simulink model "sudoku"  (R2012b)
settings: Solver=ode45  StartTime=0.0  StopTime=10.0  RelTol=1e-3
libraries: sldvlib x83
(part 1 of 4)
settings Model: Creator=roberto  LastModifiedBy=roberto

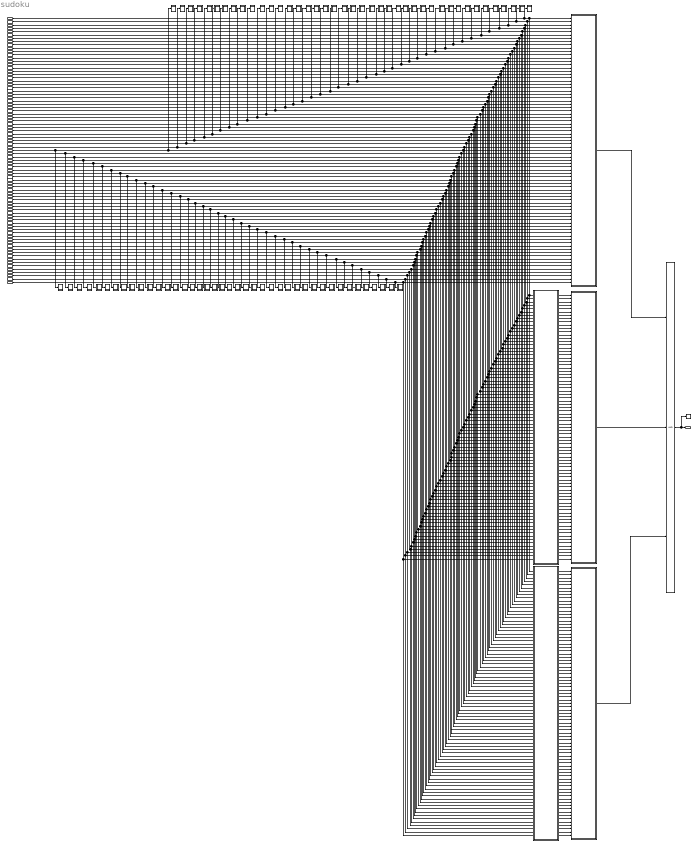
== system sudoku ==
  In1 : Inport  OutDataTypeStr=int8
  In2 : Inport  Port=2  OutDataTypeStr=int8
  In3 : Inport  Port=3  OutDataTypeStr=int8
  In4 : Inport  Port=4  OutDataTypeStr=int8
  In5 : Inport  Port=5  OutDataTypeStr=int8
  In6 : Inport  Port=6  OutDataTypeStr=int8
  In7 : Inport  Port=7  OutDataTypeStr=int8
  In8 : Inport  Port=8  OutDataTypeStr=int8
  In9 : Inport  Port=9  OutDataTypeStr=int8
  In10 : Inport  Port=10  OutDataTypeStr=int8
  In11 : Inport  Port=11  OutDataTypeStr=int8
  In12 : Inport  Port=12  OutDataTypeStr=int8
  In13 : Inport  Port=13  OutDataTypeStr=int8
  In14 : Inport  Port=14  OutDataTypeStr=int8
  In15 : Inport  Port=15  OutDataTypeStr=int8
  In16 : Inport  Port=16  OutDataTypeStr=int8
  In17 : Inport  Port=17  OutDataTypeStr=int8
  In18 : Inport  Port=18  OutDataTypeStr=int8
  In19 : Inport  Port=19  OutDataTypeStr=int8
  In20 : Inport  Port=20  OutDataTypeStr=int8
  In21 : Inport  Port=21  OutDataTypeStr=int8
  In22 : Inport  Port=22  OutDataTypeStr=int8
  In23 : Inport  Port=23  OutDataTypeStr=int8
  In24 : Inport  Port=24  OutDataTypeStr=int8
  In25 : Inport  Port=25  OutDataTypeStr=int8
  In26 : Inport  Port=26  OutDataTypeStr=int8
  In27 : Inport  Port=27  OutDataTypeStr=int8
  In28 : Inport  Port=28  OutDataTypeStr=int8
  In29 : Inport  Port=29  OutDataTypeStr=int8
  In30 : Inport  Port=30  OutDataTypeStr=int8
  In31 : Inport  Port=31  OutDataTypeStr=int8
  In32 : Inport  Port=32  OutDataTypeStr=int8
  In33 : Inport  Port=33  OutDataTypeStr=int8
  In34 : Inport  Port=34  OutDataTypeStr=int8
  In35 : Inport  Port=35  OutDataTypeStr=int8
  In36 : Inport  Port=36  OutDataTypeStr=int8
  In37 : Inport  Port=37  OutDataTypeStr=int8
  In38 : Inport  Port=38  OutDataTypeStr=int8
  In39 : Inport  Port=39  OutDataTypeStr=int8
  In40 : Inport  Port=40  OutDataTypeStr=int8
  In41 : Inport  Port=41  OutDataTypeStr=int8
  In42 : Inport  Port=42  OutDataTypeStr=int8
  In43 : Inport  Port=43  OutDataTypeStr=int8
  In44 : Inport  Port=44  OutDataTypeStr=int8
  In45 : Inport  Port=45  OutDataTypeStr=int8
  In46 : Inport  Port=46  OutDataTypeStr=int8
  In47 : Inport  Port=47  OutDataTypeStr=int8
  In48 : Inport  Port=48  OutDataTypeStr=int8
  In49 : Inport  Port=49  OutDataTypeStr=int8
  In50 : Inport  Port=50  OutDataTypeStr=int8
  In51 : Inport  Port=51  OutDataTypeStr=int8
  In52 : Inport  Port=52  OutDataTypeStr=int8
  In53 : Inport  Port=53  OutDataTypeStr=int8
  In54 : Inport  Port=54  OutDataTypeStr=int8
  In55 : Inport  Port=55  OutDataTypeStr=int8
  In56 : Inport  Port=56  OutDataTypeStr=int8
  In57 : Inport  Port=57  OutDataTypeStr=int8
  In58 : Inport  Port=58  OutDataTypeStr=int8
  In59 : Inport  Port=59  OutDataTypeStr=int8
  In60 : Inport  Port=60  OutDataTypeStr=int8
  In61 : Inport  Port=61  OutDataTypeStr=int8
  In62 : Inport  Port=62  OutDataTypeStr=int8
  In63 : Inport  Port=63  OutDataTypeStr=int8
  In64 : Inport  Port=64  OutDataTypeStr=int8
  In65 : Inport  Port=65  OutDataTypeStr=int8
  In66 : Inport  Port=66  OutDataTypeStr=int8
  In67 : Inport  Port=67  OutDataTypeStr=int8
  In68 : Inport  Port=68  OutDataTypeStr=int8
  In69 : Inport  Port=69  OutDataTypeStr=int8
  In70 : Inport  Port=70  OutDataTypeStr=int8
  In71 : Inport  Port=71  OutDataTypeStr=int8
  In72 : Inport  Port=72  OutDataTypeStr=int8
  In73 : Inport  Port=73  OutDataTypeStr=int8
  In74 : Inport  Port=74  OutDataTypeStr=int8
  In75 : Inport  Port=75  OutDataTypeStr=int8
  In76 : Inport  Port=76  OutDataTypeStr=int8
  In77 : Inport  Port=77  OutDataTypeStr=int8
  In78 : Inport  Port=78  OutDataTypeStr=int8
  In79 : Inport  Port=79  OutDataTypeStr=int8
  In80 : Inport  Port=80  OutDataTypeStr=int8
  In81 : Inport  Port=81  OutDataTypeStr=int8
  BlockRewire : Subsystem
  ColRewire : Subsystem
  Logical Operator : Logic  Inputs=3  AllPortsSameDT=off  OutDataTypeStr=boolean
  Proof Objective : sldvlib/Objectives and Constraints/Proof Objective  enabled=on  customAVTBlockType=Proof Objective  intervals=true  dispValues=on  outEnabled=on  enableStopSim=off
      settings: AttributesFormatString=%<intervals>
  Rows : Subsystem
  blocks : Subsystem
  bounds : Subsystem
  bounds1 : Subsystem
  bounds10 : Subsystem
  bounds11 : Subsystem
  bounds12 : Subsystem
  bounds13 : Subsystem
  bounds14 : Subsystem
  bounds15 : Subsystem
  bounds16 : Subsystem
  bounds17 : Subsystem
  bounds18 : Subsystem
  bounds19 : Subsystem
  bounds2 : Subsystem
  bounds20 : Subsystem
  bounds21 : Subsystem
  bounds22 : Subsystem
  bounds23 : Subsystem
  bounds24 : Subsystem
  bounds25 : Subsystem
  bounds26 : Subsystem
  bounds27 : Subsystem
  bounds28 : Subsystem
  bounds29 : Subsystem
  bounds3 : Subsystem
  bounds30 : Subsystem
  bounds31 : Subsystem
  bounds32 : Subsystem
  bounds33 : Subsystem
  bounds34 : Subsystem
  bounds35 : Subsystem
  bounds36 : Subsystem
  bounds37 : Subsystem
  bounds38 : Subsystem
  bounds39 : Subsystem
  bounds4 : Subsystem
  bounds40 : Subsystem
  bounds41 : Subsystem
  bounds42 : Subsystem
  bounds43 : Subsystem
  bounds44 : Subsystem
  bounds45 : Subsystem
  bounds46 : Subsystem
  bounds47 : Subsystem
  bounds48 : Subsystem
  bounds49 : Subsystem
  bounds5 : Subsystem
  bounds50 : Subsystem
  bounds51 : Subsystem
  bounds52 : Subsystem
  bounds53 : Subsystem
  bounds54 : Subsystem
  bounds55 : Subsystem
  bounds56 : Subsystem
  bounds57 : Subsystem
  bounds58 : Subsystem
  bounds59 : Subsystem
  bounds6 : Subsystem
  bounds60 : Subsystem
  bounds61 : Subsystem
  bounds62 : Subsystem
  bounds63 : Subsystem
  bounds64 : Subsystem
  bounds65 : Subsystem
  bounds66 : Subsystem
  bounds67 : Subsystem
  bounds68 : Subsystem
  bounds69 : Subsystem
  bounds7 : Subsystem
  bounds70 : Subsystem
  bounds71 : Subsystem
  bounds72 : Subsystem
  bounds73 : Subsystem
  bounds74 : Subsystem
  bounds75 : Subsystem
  bounds76 : Subsystem
  bounds77 : Subsystem
  bounds78 : Subsystem
  bounds79 : Subsystem
  bounds8 : Subsystem
  bounds80 : Subsystem
  bounds81 : Subsystem
  bounds9 : Subsystem
  columns : Subsystem
  Out1 : Outport
  wires:
  In2/1 -> bounds1/1(In1), BlockRewire/2(In2), ColRewire/2(In2), Rows/2(In2)
  In3/1 -> bounds2/1(In1), BlockRewire/3(In3), ColRewire/3(In3), Rows/3(In3)
  In4/1 -> bounds3/1(In1), BlockRewire/4(In4), ColRewire/4(In4), Rows/4(In4)
  In5/1 -> bounds4/1(In1), BlockRewire/5(In5), ColRewire/5(In5), Rows/5(In5)
  In6/1 -> bounds5/1(In1), BlockRewire/6(In6), ColRewire/6(In6), Rows/6(In6)
  In7/1 -> bounds6/1(In1), BlockRewire/7(In7), ColRewire/7(In7), Rows/7(In7)
  In8/1 -> bounds7/1(In1), BlockRewire/8(In8), ColRewire/8(In8), Rows/8(In8)
  In9/1 -> bounds8/1(In1), BlockRewire/9(In9), ColRewire/9(In9), Rows/9(In9)
  In10/1 -> bounds9/1(In1), BlockRewire/10(In10), ColRewire/10(In10), Rows/10(In10)
  In11/1 -> bounds10/1(In1), BlockRewire/11(In11), ColRewire/11(In11), Rows/11(In11)
  In12/1 -> bounds11/1(In1), BlockRewire/12(In12), ColRewire/12(In12), Rows/12(In12)
  In13/1 -> bounds12/1(In1), BlockRewire/13(In13), ColRewire/13(In13), Rows/13(In13)
  In14/1 -> bounds13/1(In1), BlockRewire/14(In14), ColRewire/14(In14), Rows/14(In14)
  In16/1 -> bounds15/1(In1), BlockRewire/16(In16), ColRewire/16(In16), Rows/16(In16)
  In17/1 -> bounds16/1(In1), BlockRewire/17(In17), ColRewire/17(In17), Rows/17(In17)
  In18/1 -> bounds17/1(In1), BlockRewire/18(In18), ColRewire/18(In18), Rows/18(In18)
  In19/1 -> bounds18/1(In1), BlockRewire/19(In19), ColRewire/19(In19), Rows/19(In19)
  In21/1 -> bounds20/1(In1), BlockRewire/21(In21), ColRewire/21(In21), Rows/21(In21)
  In22/1 -> bounds21/1(In1), BlockRewire/22(In22), ColRewire/22(In22), Rows/22(In22)
  In23/1 -> bounds22/1(In1), BlockRewire/23(In23), ColRewire/23(In23), Rows/23(In23)
  In24/1 -> bounds23/1(In1), BlockRewire/24(In24), ColRewire/24(In24), Rows/24(In24)
  In25/1 -> bounds24/1(In1), BlockRewire/25(In25), ColRewire/25(In25), Rows/25(In25)
  In26/1 -> bounds25/1(In1), BlockRewire/26(In26), ColRewire/26(In26), Rows/26(In26)
  In27/1 -> bounds26/1(In1), BlockRewire/27(In27), ColRewire/27(In27), Rows/27(In27)
  In28/1 -> bounds27/1(In1), BlockRewire/28(In28), ColRewire/28(In28), Rows/28(In28)
  In29/1 -> bounds28/1(In1), BlockRewire/29(In29), ColRewire/29(In29), Rows/29(In29)
  In30/1 -> bounds29/1(In1), BlockRewire/30(In30), ColRewire/30(In30), Rows/30(In30)
  In31/1 -> bounds30/1(In1), BlockRewire/31(In31), ColRewire/31(In31), Rows/31(In31)
  In33/1 -> bounds32/1(In1), BlockRewire/33(In33), ColRewire/33(In33), Rows/33(In33)
  In34/1 -> bounds33/1(In1), BlockRewire/34(In34), ColRewire/34(In34), Rows/34(In34)
  In35/1 -> bounds34/1(In1), BlockRewire/35(In35), ColRewire/35(In35), Rows/35(In35)
  In36/1 -> bounds35/1(In1), BlockRewire/36(In36), ColRewire/36(In36), Rows/36(In36)
  In38/1 -> bounds37/1(In1), BlockRewire/38(In38), ColRewire/38(In38), Rows/38(In38)
  In39/1 -> bounds38/1(In1), BlockRewire/39(In39), ColRewire/39(In39), Rows/39(In39)
  In40/1 -> bounds39/1(In1), BlockRewire/40(In40), ColRewire/40(In40), Rows/40(In40)
  In42/1 -> bounds43/1(In1), BlockRewire/42(In42), ColRewire/42(In42), Rows/42(In42)
  In43/1 -> bounds44/1(In1), BlockRewire/43(In43), ColRewire/43(In43), Rows/43(In43)
  In44/1 -> bounds45/1(In1), BlockRewire/44(In44), ColRewire/44(In44), Rows/44(In44)
  In45/1 -> bounds46/1(In1), BlockRewire/45(In45), ColRewire/45(In45), Rows/45(In45)
  In46/1 -> bounds47/1(In1), BlockRewire/46(In46), ColRewire/46(In46), Rows/46(In46)
  In47/1 -> bounds48/1(In1), BlockRewire/47(In47), ColRewire/47(In47), Rows/47(In47)
  In48/1 -> bounds49/1(In1), BlockRewire/48(In48), ColRewire/48(In48), Rows/48(In48)
  In49/1 -> bounds50/1(In1), BlockRewire/49(In49), ColRewire/49(In49), Rows/49(In49)
  In50/1 -> bounds51/1(In1), BlockRewire/50(In50), ColRewire/50(In50), Rows/50(In50)
  In51/1 -> bounds52/1(In1), BlockRewire/51(In51), ColRewire/51(In51), Rows/51(In51)
  In52/1 -> bounds53/1(In1), BlockRewire/52(In52), ColRewire/52(In52), Rows/52(In52)
  In53/1 -> bounds54/1(In1), BlockRewire/53(In53), ColRewire/53(In53), Rows/53(In53)
  In54/1 -> bounds55/1(In1), BlockRewire/54(In54), ColRewire/54(In54), Rows/54(In54)
  In55/1 -> bounds56/1(In1), BlockRewire/55(In55), ColRewire/55(In55), Rows/55(In55)
  In56/1 -> bounds57/1(In1), BlockRewire/56(In56), ColRewire/56(In56), Rows/56(In56)
  In57/1 -> bounds58/1(In1), BlockRewire/57(In57), ColRewire/57(In57), Rows/57(In57)
  In58/1 -> bounds59/1(In1), BlockRewire/58(In58), ColRewire/58(In58), Rows/58(In58)
  In59/1 -> bounds60/1(In1), BlockRewire/59(In59), ColRewire/59(In59), Rows/59(In59)
  In60/1 -> bounds61/1(In1), BlockRewire/60(In60), ColRewire/60(In60), Rows/60(In60)
  In61/1 -> bounds62/1(In1), BlockRewire/61(In61), ColRewire/61(In61), Rows/61(In61)
  In62/1 -> bounds63/1(In1), BlockRewire/62(In62), ColRewire/62(In62), Rows/62(In62)
  In63/1 -> bounds64/1(In1), ColRewire/63(In63), BlockRewire/63(In63), Rows/63(In63)
  In64/1 -> bounds65/1(In1), BlockRewire/64(In64), ColRewire/64(In64), Rows/64(In64)
  In66/1 -> bounds67/1(In1), BlockRewire/66(In66), ColRewire/66(In66), Rows/66(In66)
  In68/1 -> bounds69/1(In1), BlockRewire/68(In68), ColRewire/68(In68), Rows/68(In68)
  In70/1 -> bounds71/1(In1), BlockRewire/70(In70), ColRewire/70(In70), Rows/70(In70)
  In71/1 -> bounds72/1(In1), BlockRewire/71(In71), ColRewire/71(In71), Rows/71(In71)
  In72/1 -> bounds73/1(In1), BlockRewire/72(In72), ColRewire/72(In72), Rows/72(In72)
  In74/1 -> bounds75/1(In1), BlockRewire/74(In74), ColRewire/74(In74), Rows/74(In74)
  In75/1 -> bounds76/1(In1), BlockRewire/75(In75), ColRewire/75(In75), Rows/75(In75)
  In76/1 -> bounds77/1(In1), BlockRewire/76(In76), ColRewire/76(In76), Rows/76(In76)
  In77/1 -> bounds78/1(In1), BlockRewire/77(In77), ColRewire/77(In77), Rows/77(In77)
  In78/1 -> bounds79/1(In1), BlockRewire/78(In78), ColRewire/78(In78), Rows/78(In78)
  In79/1 -> bounds80/1(In1), BlockRewire/79(In79), ColRewire/79(In79), Rows/79(In79)
  In80/1 -> bounds81/1(In1), BlockRewire/80(In80), ColRewire/80(In80), Rows/80(In80)
  In81/1 -> bounds41/1(In1), BlockRewire/81(In81), ColRewire/81(In81), Rows/81(In81)
  In69/1 -> bounds70/1(In1), BlockRewire/69(In69), ColRewire/69(In69), Rows/69(In69)
  In73/1 -> bounds74/1(In1), BlockRewire/73(In73), ColRewire/73(In73), Rows/73(In73)
  ColRewire/1(Out1) -> columns/1(In1)
  ColRewire/2(Out2) -> columns/2(In2)
  ColRewire/3(Out3) -> columns/3(In3)
  ColRewire/4(Out4) -> columns/4(In4)
  ColRewire/5(Out5) -> columns/5(In5)
  ColRewire/6(Out6) -> columns/6(In6)
  ColRewire/7(Out7) -> columns/7(In7)
  ColRewire/8(Out8) -> columns/8(In8)
  ColRewire/9(Out9) -> columns/9(In9)
  ColRewire/10(Out10) -> columns/10(In10)
  ColRewire/11(Out11) -> columns/11(In11)
  ColRewire/12(Out12) -> columns/12(In12)
  ColRewire/13(Out13) -> columns/13(In13)
  ColRewire/14(Out14) -> columns/14(In14)
  ColRewire/15(Out15) -> columns/15(In15)
  ColRewire/16(Out16) -> columns/16(In16)
  ColRewire/17(Out17) -> columns/17(In17)
  ColRewire/18(Out18) -> columns/18(In18)
  ColRewire/19(Out19) -> columns/19(In19)
  ColRewire/20(Out20) -> columns/20(In20)
  ColRewire/21(Out21) -> columns/21(In21)
  ColRewire/22(Out22) -> columns/22(In22)
  ColRewire/23(Out23) -> columns/23(In23)
  ColRewire/24(Out24) -> columns/24(In24)
  ColRewire/25(Out25) -> columns/25(In25)
  ColRewire/26(Out26) -> columns/26(In26)
  ColRewire/27(Out27) -> columns/27(In27)
  ColRewire/28(Out28) -> columns/28(In28)
  ColRewire/29(Out29) -> columns/29(In29)
  ColRewire/30(Out30) -> columns/30(In30)
  ColRewire/31(Out31) -> columns/31(In31)
  ColRewire/32(Out32) -> columns/32(In32)
  ColRewire/33(Out33) -> columns/33(In33)
  ColRewire/34(Out34) -> columns/34(In34)
  ColRewire/35(Out35) -> columns/35(In35)
  ColRewire/36(Out36) -> columns/36(In36)
  ColRewire/37(Out37) -> columns/37(In37)
  ColRewire/38(Out38) -> columns/38(In38)
  ColRewire/39(Out39) -> columns/39(In39)
  ColRewire/40(Out40) -> columns/40(In40)
  ColRewire/41(Out41) -> columns/41(In41)
  ColRewire/42(Out42) -> columns/42(In42)
  ColRewire/43(Out43) -> columns/43(In43)
  ColRewire/44(Out44) -> columns/44(In44)
  ColRewire/45(Out45) -> columns/45(In45)
  ColRewire/46(Out46) -> columns/46(In46)
  ColRewire/47(Out47) -> columns/47(In47)
  ColRewire/48(Out48) -> columns/48(In48)
  ColRewire/49(Out49) -> columns/49(In49)
  ColRewire/50(Out50) -> columns/50(In50)
  ColRewire/51(Out51) -> columns/51(In51)
  ColRewire/52(Out52) -> columns/52(In52)
  ColRewire/53(Out53) -> columns/53(In53)
  ColRewire/54(Out54) -> columns/54(In54)
  ColRewire/55(Out55) -> columns/55(In55)
  ColRewire/56(Out56) -> columns/56(In56)
  ColRewire/57(Out57) -> columns/57(In57)
  ColRewire/58(Out58) -> columns/58(In58)
  ColRewire/59(Out59) -> columns/59(In59)
  ColRewire/60(Out60) -> columns/60(In60)
  ColRewire/61(Out61) -> columns/61(In61)
  ColRewire/62(Out62) -> columns/62(In62)
  ColRewire/63(Out63) -> columns/63(In63)
  ColRewire/64(Out64) -> columns/64(In64)
  ColRewire/65(Out65) -> columns/65(In65)
  ColRewire/66(Out66) -> columns/66(In66)
  ColRewire/67(Out67) -> columns/67(In67)
  ColRewire/68(Out68) -> columns/68(In68)
  ColRewire/70(Out70) -> columns/70(In70)
  ColRewire/71(Out71) -> columns/71(In71)
  ColRewire/72(Out72) -> columns/72(In72)
  ColRewire/74(Out74) -> columns/74(In74)
  ColRewire/75(Out75) -> columns/75(In75)
  ColRewire/76(Out76) -> columns/76(In76)
  ColRewire/77(Out77) -> columns/77(In77)
  ColRewire/78(Out78) -> columns/78(In78)
  ColRewire/79(Out79) -> columns/79(In79)
  ColRewire/80(Out80) -> columns/80(In80)
  ColRewire/81(Out81) -> columns/81(In81)
  ColRewire/69(Out69) -> columns/69(In69)
  ColRewire/73(Out73) -> columns/73(In73)
  BlockRewire/1(Out1) -> blocks/1(In1)
  BlockRewire/2(Out10) -> blocks/2(In2)
  BlockRewire/3(Out19) -> blocks/3(In3)
  BlockRewire/4(Out2) -> blocks/4(In4)
  BlockRewire/5(Out11) -> blocks/5(In5)
  BlockRewire/6(Out20) -> blocks/6(In6)
  BlockRewire/7(Out3) -> blocks/7(In7)
  BlockRewire/8(Out12) -> blocks/8(In8)
  BlockRewire/9(Out21) -> blocks/9(In9)
  BlockRewire/10(Out28) -> blocks/10(In10)
  BlockRewire/11(Out37) -> blocks/11(In11)
  BlockRewire/12(Out46) -> blocks/12(In12)
  BlockRewire/13(Out29) -> blocks/13(In13)
  BlockRewire/15(Out47) -> blocks/15(In15)
  BlockRewire/16(Out30) -> blocks/16(In16)
  BlockRewire/17(Out39) -> blocks/17(In17)
  BlockRewire/18(Out48) -> blocks/18(In18)
  BlockRewire/19(Out55) -> blocks/19(In19)
  BlockRewire/20(Out64) -> blocks/20(In20)
  BlockRewire/21(Out73) -> blocks/21(In21)
  BlockRewire/22(Out56) -> blocks/22(In22)
  BlockRewire/23(Out65) -> blocks/23(In23)
  BlockRewire/24(Out74) -> blocks/24(In24)
  BlockRewire/25(Out57) -> blocks/25(In25)
  BlockRewire/26(Out66) -> blocks/26(In26)
  BlockRewire/27(Out75) -> blocks/27(In27)
  BlockRewire/28(Out4) -> blocks/28(In28)
  BlockRewire/29(Out13) -> blocks/29(In29)
  BlockRewire/30(Out22) -> blocks/30(In30)
  BlockRewire/31(Out5) -> blocks/31(In31)
  BlockRewire/32(Out14) -> blocks/32(In32)
  BlockRewire/33(Out23) -> blocks/33(In33)
  BlockRewire/34(Out6) -> blocks/34(In34)
  BlockRewire/35(Out15) -> blocks/35(In35)
  BlockRewire/36(Out24) -> blocks/36(In36)
  BlockRewire/37(Out31) -> blocks/37(In37)
  BlockRewire/38(Out40) -> blocks/38(In38)
  BlockRewire/39(Out49) -> blocks/39(In39)
  BlockRewire/40(Out32) -> blocks/40(In40)
  BlockRewire/41(Out41) -> blocks/41(In41)
  BlockRewire/42(Out50) -> blocks/42(In42)
  BlockRewire/43(Out33) -> blocks/43(In43)
  BlockRewire/44(Out42) -> blocks/44(In44)
  BlockRewire/45(Out51) -> blocks/45(In45)
  BlockRewire/46(Out58) -> blocks/46(In46)
  BlockRewire/47(Out67) -> blocks/47(In47)
  BlockRewire/48(Out76) -> blocks/48(In48)
  BlockRewire/49(Out59) -> blocks/49(In49)
  BlockRewire/50(Out68) -> blocks/50(In50)
  BlockRewire/51(Out77) -> blocks/51(In51)
  BlockRewire/52(Out60) -> blocks/52(In52)
  BlockRewire/53(Out69) -> blocks/53(In53)
  BlockRewire/54(Out78) -> blocks/54(In54)
  BlockRewire/55(Out7) -> blocks/55(In55)
  BlockRewire/56(Out16) -> blocks/56(In56)
  BlockRewire/57(Out25) -> blocks/57(In57)
  BlockRewire/58(Out8) -> blocks/58(In58)
  BlockRewire/59(Out17) -> blocks/59(In59)
  BlockRewire/60(Out26) -> blocks/60(In60)
  BlockRewire/61(Out9) -> blocks/61(In61)
  BlockRewire/62(Out18) -> blocks/62(In62)
  BlockRewire/63(Out27) -> blocks/63(In63)
  BlockRewire/64(Out34) -> blocks/64(In64)
  BlockRewire/65(Out43) -> blocks/65(In65)
  BlockRewire/66(Out52) -> blocks/66(In66)
  BlockRewire/67(Out35) -> blocks/67(In67)
  BlockRewire/68(Out44) -> blocks/68(In68)
  BlockRewire/69(Out53) -> blocks/69(In69)
  BlockRewire/70(Out36) -> blocks/70(In70)
  BlockRewire/71(Out45) -> blocks/71(In71)
  BlockRewire/72(Out54) -> blocks/72(In72)
  BlockRewire/73(Out61) -> blocks/73(In73)
  BlockRewire/74(Out70) -> blocks/74(In74)
  BlockRewire/75(Out79) -> blocks/75(In75)
  BlockRewire/76(Out62) -> blocks/76(In76)
  BlockRewire/77(Out71) -> blocks/77(In77)
  BlockRewire/78(Out80) -> blocks/78(In78)
  BlockRewire/79(Out63) -> blocks/79(In79)
  BlockRewire/80(Out72) -> blocks/80(In80)
  BlockRewire/81(Out81) -> blocks/81(In81)
  In15/1 -> bounds14/1(In1), BlockRewire/15(In15), ColRewire/15(In15), Rows/15(In15)
  In32/1 -> bounds31/1(In1), BlockRewire/32(In32), ColRewire/32(In32), Rows/32(In32)
  In37/1 -> bounds36/1(In1), BlockRewire/37(In37), ColRewire/37(In37), Rows/37(In37)
  In41/1 -> bounds42/1(In1), bounds40/1(In1), BlockRewire/41(In41), ColRewire/41(In41), Rows/41(In41)
  In65/1 -> bounds66/1(In1), ColRewire/65(In65), BlockRewire/65(In65), Rows/65(In65)
  BlockRewire/14(Out38) -> blocks/14(In14)
  In1/1 -> bounds/1(In1), BlockRewire/1(In1), ColRewire/1(In1), Rows/1(In1)
  In20/1 -> bounds19/1(In1), BlockRewire/20(In20), ColRewire/20(In20), Rows/20(In20)
  In67/1 -> bounds68/1(In1), BlockRewire/67(In67), ColRewire/67(In67), Rows/67(In67)
  Rows/1(Out1) -> Logical Operator/1
  columns/1(Out1) -> Logical Operator/2
  blocks/1(Out1) -> Logical Operator/3
  Logical Operator/1 -> Proof Objective/1, Out1/1

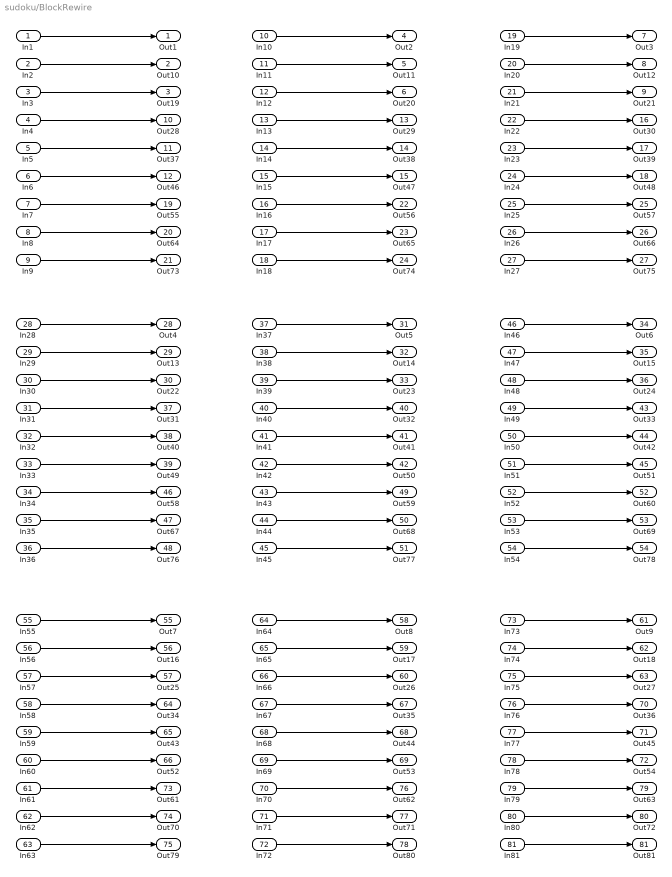
== system sudoku/BlockRewire ==
  In1 : Inport
  In2 : Inport  Port=2
  In3 : Inport  Port=3
  In4 : Inport  Port=4
  In5 : Inport  Port=5
  In6 : Inport  Port=6
  In7 : Inport  Port=7
  In8 : Inport  Port=8
  In9 : Inport  Port=9
  In10 : Inport  Port=10
  In11 : Inport  Port=11
  In12 : Inport  Port=12
  In13 : Inport  Port=13
  In14 : Inport  Port=14
  In15 : Inport  Port=15
  In16 : Inport  Port=16
  In17 : Inport  Port=17
  In18 : Inport  Port=18
  In19 : Inport  Port=19
  In20 : Inport  Port=20
  In21 : Inport  Port=21
  In22 : Inport  Port=22
  In23 : Inport  Port=23
  In24 : Inport  Port=24
  In25 : Inport  Port=25
  In26 : Inport  Port=26
  In27 : Inport  Port=27
  In28 : Inport  Port=28
  In29 : Inport  Port=29
  In30 : Inport  Port=30
  In31 : Inport  Port=31
  In32 : Inport  Port=32
  In33 : Inport  Port=33
  In34 : Inport  Port=34
  In35 : Inport  Port=35
  In36 : Inport  Port=36
  In37 : Inport  Port=37
  In38 : Inport  Port=38
  In39 : Inport  Port=39
  In40 : Inport  Port=40
  In41 : Inport  Port=41
  In42 : Inport  Port=42
  In43 : Inport  Port=43
  In44 : Inport  Port=44
  In45 : Inport  Port=45
  In46 : Inport  Port=46
  In47 : Inport  Port=47
  In48 : Inport  Port=48
  In49 : Inport  Port=49
  In50 : Inport  Port=50
  In51 : Inport  Port=51
  In52 : Inport  Port=52
  In53 : Inport  Port=53
  In54 : Inport  Port=54
  In55 : Inport  Port=55
  In56 : Inport  Port=56
  In57 : Inport  Port=57
  In58 : Inport  Port=58
  In59 : Inport  Port=59
  In60 : Inport  Port=60
  In61 : Inport  Port=61
  In62 : Inport  Port=62
  In63 : Inport  Port=63
  In64 : Inport  Port=64
  In65 : Inport  Port=65
  In66 : Inport  Port=66
  In67 : Inport  Port=67
  In68 : Inport  Port=68
  In69 : Inport  Port=69
  In70 : Inport  Port=70
  In71 : Inport  Port=71
  In72 : Inport  Port=72
  In73 : Inport  Port=73
  In74 : Inport  Port=74
  In75 : Inport  Port=75
  In76 : Inport  Port=76
  In77 : Inport  Port=77
  In78 : Inport  Port=78
  In79 : Inport  Port=79
  In80 : Inport  Port=80
  In81 : Inport  Port=81
  Out1 : Outport
  Out10 : Outport  Port=2
  Out19 : Outport  Port=3
  Out2 : Outport  Port=4
  Out11 : Outport  Port=5
  Out20 : Outport  Port=6
  Out3 : Outport  Port=7
  Out12 : Outport  Port=8
  Out21 : Outport  Port=9
  Out28 : Outport  Port=10
  Out37 : Outport  Port=11
  Out46 : Outport  Port=12
  Out29 : Outport  Port=13
  Out38 : Outport  Port=14
  Out47 : Outport  Port=15
  Out30 : Outport  Port=16
  Out39 : Outport  Port=17
  Out48 : Outport  Port=18
  Out55 : Outport  Port=19
  Out64 : Outport  Port=20
  Out73 : Outport  Port=21
  Out56 : Outport  Port=22
  Out65 : Outport  Port=23
  Out74 : Outport  Port=24
  Out57 : Outport  Port=25
  Out66 : Outport  Port=26
  Out75 : Outport  Port=27
  Out4 : Outport  Port=28
  Out13 : Outport  Port=29
  Out22 : Outport  Port=30
  Out5 : Outport  Port=31
  Out14 : Outport  Port=32
  Out23 : Outport  Port=33
  Out6 : Outport  Port=34
  Out15 : Outport  Port=35
  Out24 : Outport  Port=36
  Out31 : Outport  Port=37
  Out40 : Outport  Port=38
  Out49 : Outport  Port=39
  Out32 : Outport  Port=40
  Out41 : Outport  Port=41
  Out50 : Outport  Port=42
  Out33 : Outport  Port=43
  Out42 : Outport  Port=44
  Out51 : Outport  Port=45
  Out58 : Outport  Port=46
  Out67 : Outport  Port=47
  Out76 : Outport  Port=48
  Out59 : Outport  Port=49
  Out68 : Outport  Port=50
  Out77 : Outport  Port=51
  Out60 : Outport  Port=52
  Out69 : Outport  Port=53
  Out78 : Outport  Port=54
  Out7 : Outport  Port=55
  Out16 : Outport  Port=56
  Out25 : Outport  Port=57
  Out8 : Outport  Port=58
  Out17 : Outport  Port=59
  Out26 : Outport  Port=60
  Out9 : Outport  Port=61
  Out18 : Outport  Port=62
  Out27 : Outport  Port=63
  Out34 : Outport  Port=64
  Out43 : Outport  Port=65
  Out52 : Outport  Port=66
  Out35 : Outport  Port=67
  Out44 : Outport  Port=68
  Out53 : Outport  Port=69
  Out36 : Outport  Port=70
  Out45 : Outport  Port=71
  Out54 : Outport  Port=72
  Out61 : Outport  Port=73
  Out70 : Outport  Port=74
  Out79 : Outport  Port=75
  Out62 : Outport  Port=76
  Out71 : Outport  Port=77
  Out80 : Outport  Port=78
  Out63 : Outport  Port=79
  Out72 : Outport  Port=80
  Out81 : Outport  Port=81
  wires:
  In1/1 -> Out1/1
  In10/1 -> Out2/1
  In19/1 -> Out3/1
  In2/1 -> Out10/1
  In3/1 -> Out19/1
  In4/1 -> Out28/1
  In5/1 -> Out37/1
  In6/1 -> Out46/1
  In7/1 -> Out55/1
  In8/1 -> Out64/1
  In9/1 -> Out73/1
  In11/1 -> Out11/1
  In12/1 -> Out20/1
  In13/1 -> Out29/1
  In14/1 -> Out38/1
  In15/1 -> Out47/1
  In16/1 -> Out56/1
  In17/1 -> Out65/1
  In18/1 -> Out74/1
  In20/1 -> Out12/1
  In21/1 -> Out21/1
  In22/1 -> Out30/1
  In23/1 -> Out39/1
  In24/1 -> Out48/1
  In25/1 -> Out57/1
  In26/1 -> Out66/1
  In27/1 -> Out75/1
  In28/1 -> Out4/1
  In29/1 -> Out13/1
  In37/1 -> Out5/1
  In38/1 -> Out14/1
  In46/1 -> Out6/1
  In47/1 -> Out15/1
  In55/1 -> Out7/1
  In56/1 -> Out16/1
  In64/1 -> Out8/1
  In65/1 -> Out17/1
  In73/1 -> Out9/1
  In74/1 -> Out18/1
  In30/1 -> Out22/1
  In31/1 -> Out31/1
  In32/1 -> Out40/1
  In39/1 -> Out23/1
  In40/1 -> Out32/1
  In41/1 -> Out41/1
  In48/1 -> Out24/1
  In49/1 -> Out33/1
  In57/1 -> Out25/1
  In58/1 -> Out34/1
  In66/1 -> Out26/1
  In67/1 -> Out35/1
  In75/1 -> Out27/1
  In76/1 -> Out36/1
  In33/1 -> Out49/1
  In34/1 -> Out58/1
  In35/1 -> Out67/1
  In36/1 -> Out76/1
  In42/1 -> Out50/1
  In43/1 -> Out59/1
  In44/1 -> Out68/1
  In45/1 -> Out77/1
  In50/1 -> Out42/1
  In51/1 -> Out51/1
  In52/1 -> Out60/1
  In53/1 -> Out69/1
  In54/1 -> Out78/1
  In59/1 -> Out43/1
  In60/1 -> Out52/1
  In61/1 -> Out61/1
  In62/1 -> Out70/1
  In63/1 -> Out79/1
  In68/1 -> Out44/1
  In69/1 -> Out53/1
  In70/1 -> Out62/1
  In71/1 -> Out71/1
  In72/1 -> Out80/1
  In77/1 -> Out45/1
  In78/1 -> Out54/1
  In79/1 -> Out63/1
  In80/1 -> Out72/1
  In81/1 -> Out81/1

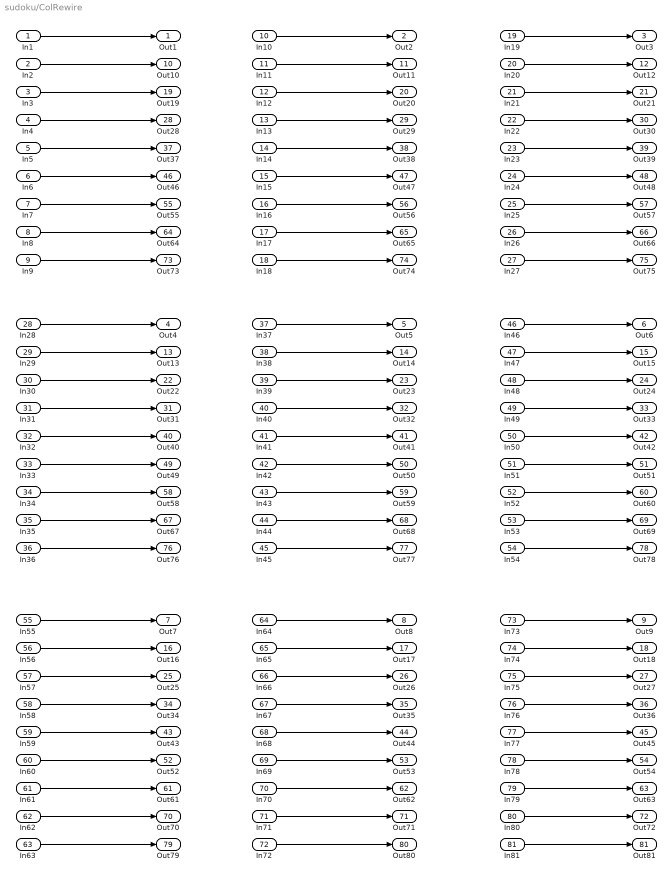
== system sudoku/ColRewire ==
  In1 : Inport
  In2 : Inport  Port=2
  In3 : Inport  Port=3
  In4 : Inport  Port=4
  In5 : Inport  Port=5
  In6 : Inport  Port=6
  In7 : Inport  Port=7
  In8 : Inport  Port=8
  In9 : Inport  Port=9
  In10 : Inport  Port=10
  In11 : Inport  Port=11
  In12 : Inport  Port=12
  In13 : Inport  Port=13
  In14 : Inport  Port=14
  In15 : Inport  Port=15
  In16 : Inport  Port=16
  In17 : Inport  Port=17
  In18 : Inport  Port=18
  In19 : Inport  Port=19
  In20 : Inport  Port=20
  In21 : Inport  Port=21
  In22 : Inport  Port=22
  In23 : Inport  Port=23
  In24 : Inport  Port=24
  In25 : Inport  Port=25
  In26 : Inport  Port=26
  In27 : Inport  Port=27
  In28 : Inport  Port=28
  In29 : Inport  Port=29
  In30 : Inport  Port=30
  In31 : Inport  Port=31
  In32 : Inport  Port=32
  In33 : Inport  Port=33
  In34 : Inport  Port=34
  In35 : Inport  Port=35
  In36 : Inport  Port=36
  In37 : Inport  Port=37
  In38 : Inport  Port=38
  In39 : Inport  Port=39
  In40 : Inport  Port=40
  In41 : Inport  Port=41
  In42 : Inport  Port=42
  In43 : Inport  Port=43
  In44 : Inport  Port=44
  In45 : Inport  Port=45
  In46 : Inport  Port=46
  In47 : Inport  Port=47
  In48 : Inport  Port=48
  In49 : Inport  Port=49
  In50 : Inport  Port=50
  In51 : Inport  Port=51
  In52 : Inport  Port=52
  In53 : Inport  Port=53
  In54 : Inport  Port=54
  In55 : Inport  Port=55
  In56 : Inport  Port=56
  In57 : Inport  Port=57
  In58 : Inport  Port=58
  In59 : Inport  Port=59
  In60 : Inport  Port=60
  In61 : Inport  Port=61
  In62 : Inport  Port=62
  In63 : Inport  Port=63
  In64 : Inport  Port=64
  In65 : Inport  Port=65
  In66 : Inport  Port=66
  In67 : Inport  Port=67
  In68 : Inport  Port=68
  In69 : Inport  Port=69
  In70 : Inport  Port=70
  In71 : Inport  Port=71
  In72 : Inport  Port=72
  In73 : Inport  Port=73
  In74 : Inport  Port=74
  In75 : Inport  Port=75
  In76 : Inport  Port=76
  In77 : Inport  Port=77
  In78 : Inport  Port=78
  In79 : Inport  Port=79
  In80 : Inport  Port=80
  In81 : Inport  Port=81
  Out1 : Outport
  Out2 : Outport  Port=2
  Out3 : Outport  Port=3
  Out4 : Outport  Port=4
  Out5 : Outport  Port=5
  Out6 : Outport  Port=6
  Out7 : Outport  Port=7
  Out8 : Outport  Port=8
  Out9 : Outport  Port=9
  Out10 : Outport  Port=10
  Out11 : Outport  Port=11
  Out12 : Outport  Port=12
  Out13 : Outport  Port=13
  Out14 : Outport  Port=14
  Out15 : Outport  Port=15
  Out16 : Outport  Port=16
  Out17 : Outport  Port=17
  Out18 : Outport  Port=18
  Out19 : Outport  Port=19
  Out20 : Outport  Port=20
  Out21 : Outport  Port=21
  Out22 : Outport  Port=22
  Out23 : Outport  Port=23
  Out24 : Outport  Port=24
  Out25 : Outport  Port=25
  Out26 : Outport  Port=26
  Out27 : Outport  Port=27
  Out28 : Outport  Port=28
  Out29 : Outport  Port=29
  Out30 : Outport  Port=30
  Out31 : Outport  Port=31
  Out32 : Outport  Port=32
  Out33 : Outport  Port=33
  Out34 : Outport  Port=34
  Out35 : Outport  Port=35
  Out36 : Outport  Port=36
  Out37 : Outport  Port=37
  Out38 : Outport  Port=38
  Out39 : Outport  Port=39
  Out40 : Outport  Port=40
  Out41 : Outport  Port=41
  Out42 : Outport  Port=42
  Out43 : Outport  Port=43
  Out44 : Outport  Port=44
  Out45 : Outport  Port=45
  Out46 : Outport  Port=46
  Out47 : Outport  Port=47
  Out48 : Outport  Port=48
  Out49 : Outport  Port=49
  Out50 : Outport  Port=50
  Out51 : Outport  Port=51
  Out52 : Outport  Port=52
  Out53 : Outport  Port=53
  Out54 : Outport  Port=54
  Out55 : Outport  Port=55
  Out56 : Outport  Port=56
  Out57 : Outport  Port=57
  Out58 : Outport  Port=58
  Out59 : Outport  Port=59
  Out60 : Outport  Port=60
  Out61 : Outport  Port=61
  Out62 : Outport  Port=62
  Out63 : Outport  Port=63
  Out64 : Outport  Port=64
  Out65 : Outport  Port=65
  Out66 : Outport  Port=66
  Out67 : Outport  Port=67
  Out68 : Outport  Port=68
  Out69 : Outport  Port=69
  Out70 : Outport  Port=70
  Out71 : Outport  Port=71
  Out72 : Outport  Port=72
  Out73 : Outport  Port=73
  Out74 : Outport  Port=74
  Out75 : Outport  Port=75
  Out76 : Outport  Port=76
  Out77 : Outport  Port=77
  Out78 : Outport  Port=78
  Out79 : Outport  Port=79
  Out80 : Outport  Port=80
  Out81 : Outport  Port=81
  wires:
  In1/1 -> Out1/1
  In10/1 -> Out2/1
  In19/1 -> Out3/1
  In2/1 -> Out10/1
  In3/1 -> Out19/1
  In4/1 -> Out28/1
  In5/1 -> Out37/1
  In6/1 -> Out46/1
  In7/1 -> Out55/1
  In8/1 -> Out64/1
  In9/1 -> Out73/1
  In11/1 -> Out11/1
  In12/1 -> Out20/1
  In13/1 -> Out29/1
  In14/1 -> Out38/1
  In15/1 -> Out47/1
  In16/1 -> Out56/1
  In17/1 -> Out65/1
  In18/1 -> Out74/1
  In20/1 -> Out12/1
  In21/1 -> Out21/1
  In22/1 -> Out30/1
  In23/1 -> Out39/1
  In24/1 -> Out48/1
  In25/1 -> Out57/1
  In26/1 -> Out66/1
  In27/1 -> Out75/1
  In28/1 -> Out4/1
  In29/1 -> Out13/1
  In37/1 -> Out5/1
  In38/1 -> Out14/1
  In46/1 -> Out6/1
  In47/1 -> Out15/1
  In55/1 -> Out7/1
  In56/1 -> Out16/1
  In64/1 -> Out8/1
  In65/1 -> Out17/1
  In73/1 -> Out9/1
  In74/1 -> Out18/1
  In30/1 -> Out22/1
  In31/1 -> Out31/1
  In32/1 -> Out40/1
  In39/1 -> Out23/1
  In40/1 -> Out32/1
  In41/1 -> Out41/1
  In48/1 -> Out24/1
  In49/1 -> Out33/1
  In57/1 -> Out25/1
  In58/1 -> Out34/1
  In66/1 -> Out26/1
  In67/1 -> Out35/1
  In75/1 -> Out27/1
  In76/1 -> Out36/1
  In33/1 -> Out49/1
  In34/1 -> Out58/1
  In35/1 -> Out67/1
  In36/1 -> Out76/1
  In42/1 -> Out50/1
  In43/1 -> Out59/1
  In44/1 -> Out68/1
  In45/1 -> Out77/1
  In50/1 -> Out42/1
  In51/1 -> Out51/1
  In52/1 -> Out60/1
  In53/1 -> Out69/1
  In54/1 -> Out78/1
  In59/1 -> Out43/1
  In60/1 -> Out52/1
  In61/1 -> Out61/1
  In62/1 -> Out70/1
  In63/1 -> Out79/1
  In68/1 -> Out44/1
  In69/1 -> Out53/1
  In70/1 -> Out62/1
  In71/1 -> Out71/1
  In72/1 -> Out80/1
  In77/1 -> Out45/1
  In78/1 -> Out54/1
  In79/1 -> Out63/1
  In80/1 -> Out72/1
  In81/1 -> Out81/1

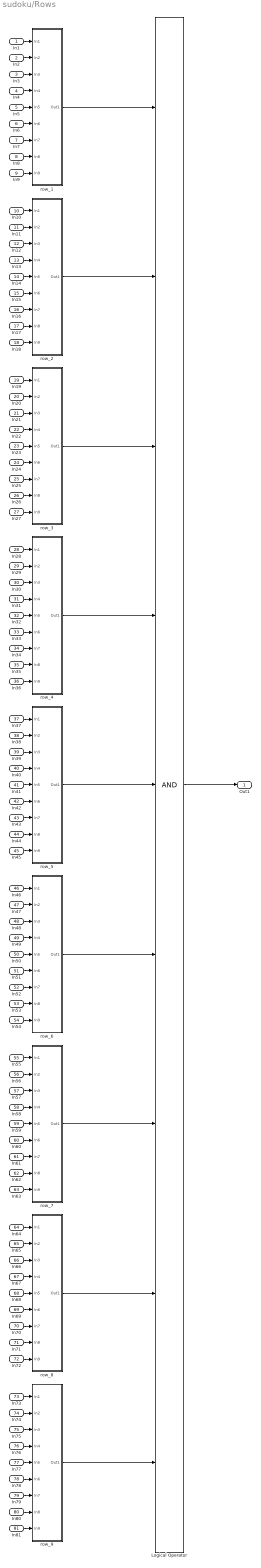
== system sudoku/Rows ==
  In1 : Inport
  In2 : Inport  Port=2
  In3 : Inport  Port=3
  In4 : Inport  Port=4
  In5 : Inport  Port=5
  In6 : Inport  Port=6
  In7 : Inport  Port=7
  In8 : Inport  Port=8
  In9 : Inport  Port=9
  In10 : Inport  Port=10
  In11 : Inport  Port=11
  In12 : Inport  Port=12
  In13 : Inport  Port=13
  In14 : Inport  Port=14
  In15 : Inport  Port=15
  In16 : Inport  Port=16
  In17 : Inport  Port=17
  In18 : Inport  Port=18
  In19 : Inport  Port=19
  In20 : Inport  Port=20
  In21 : Inport  Port=21
  In22 : Inport  Port=22
  In23 : Inport  Port=23
  In24 : Inport  Port=24
  In25 : Inport  Port=25
  In26 : Inport  Port=26
  In27 : Inport  Port=27
  In28 : Inport  Port=28
  In29 : Inport  Port=29
  In30 : Inport  Port=30
  In31 : Inport  Port=31
  In32 : Inport  Port=32
  In33 : Inport  Port=33
  In34 : Inport  Port=34
  In35 : Inport  Port=35
  In36 : Inport  Port=36
  In37 : Inport  Port=37
  In38 : Inport  Port=38
  In39 : Inport  Port=39
  In40 : Inport  Port=40
  In41 : Inport  Port=41
  In42 : Inport  Port=42
  In43 : Inport  Port=43
  In44 : Inport  Port=44
  In45 : Inport  Port=45
  In46 : Inport  Port=46
  In47 : Inport  Port=47
  In48 : Inport  Port=48
  In49 : Inport  Port=49
  In50 : Inport  Port=50
  In51 : Inport  Port=51
  In52 : Inport  Port=52
  In53 : Inport  Port=53
  In54 : Inport  Port=54
  In55 : Inport  Port=55
  In56 : Inport  Port=56
  In57 : Inport  Port=57
  In58 : Inport  Port=58
  In59 : Inport  Port=59
  In60 : Inport  Port=60
  In61 : Inport  Port=61
  In62 : Inport  Port=62
  In63 : Inport  Port=63
  In64 : Inport  Port=64
  In65 : Inport  Port=65
  In66 : Inport  Port=66
  In67 : Inport  Port=67
  In68 : Inport  Port=68
  In69 : Inport  Port=69
  In70 : Inport  Port=70
  In71 : Inport  Port=71
  In72 : Inport  Port=72
  In73 : Inport  Port=73
  In74 : Inport  Port=74
  In75 : Inport  Port=75
  In76 : Inport  Port=76
  In77 : Inport  Port=77
  In78 : Inport  Port=78
  In79 : Inport  Port=79
  In80 : Inport  Port=80
  In81 : Inport  Port=81
  Logical Operator : Logic  Inputs=9  AllPortsSameDT=off  OutDataTypeStr=boolean
  row_1 : Subsystem
  row_2 : Subsystem
  row_3 : Subsystem
  row_4 : Subsystem
  row_5 : Subsystem
  row_6 : Subsystem
  row_7 : Subsystem
  row_8 : Subsystem
  row_9 : Subsystem
  Out1 : Outport
  wires:
  In13/1 -> row_2/4(In4)
  In10/1 -> row_2/1(In1)
  In14/1 -> row_2/5(In5)
  In16/1 -> row_2/7(In7)
  In18/1 -> row_2/9(In9)
  In12/1 -> row_2/3(In3)
  In63/1 -> row_7/9(In9)
  In62/1 -> row_7/8(In8)
  In17/1 -> row_2/8(In8)
  In11/1 -> row_2/2(In2)
  In15/1 -> row_2/6(In6)
  In47/1 -> row_6/2(In2)
  In48/1 -> row_6/3(In3)
  In59/1 -> row_7/5(In5)
  In60/1 -> row_7/6(In6)
  In56/1 -> row_7/2(In2)
  In57/1 -> row_7/3(In3)
  In58/1 -> row_7/4(In4)
  In55/1 -> row_7/1(In1)
  In61/1 -> row_7/7(In7)
  In32/1 -> row_4/5(In5)
  In33/1 -> row_4/6(In6)
  In28/1 -> row_4/1(In1)
  In2/1 -> row_1/2(In2)
  In4/1 -> row_1/4(In4)
  In8/1 -> row_1/8(In8)
  In9/1 -> row_1/9(In9)
  In35/1 -> row_4/8(In8)
  In34/1 -> row_4/7(In7)
  In1/1 -> row_1/1(In1)
  In6/1 -> row_1/6(In6)
  In7/1 -> row_1/7(In7)
  In49/1 -> row_6/4(In4)
  In50/1 -> row_6/5(In5)
  In51/1 -> row_6/6(In6)
  In52/1 -> row_6/7(In7)
  In53/1 -> row_6/8(In8)
  In3/1 -> row_1/3(In3)
  In54/1 -> row_6/9(In9)
  In37/1 -> row_5/1(In1)
  In46/1 -> row_6/1(In1)
  In5/1 -> row_1/5(In5)
  In38/1 -> row_5/2(In2)
  In39/1 -> row_5/3(In3)
  In36/1 -> row_4/9(In9)
  In29/1 -> row_4/2(In2)
  In30/1 -> row_4/3(In3)
  In31/1 -> row_4/4(In4)
  In65/1 -> row_8/2(In2)
  In43/1 -> row_5/7(In7)
  In72/1 -> row_8/9(In9)
  In69/1 -> row_8/6(In6)
  In20/1 -> row_3/2(In2)
  In25/1 -> row_3/7(In7)
  In80/1 -> row_9/8(In8)
  In42/1 -> row_5/6(In6)
  In22/1 -> row_3/4(In4)
  In45/1 -> row_5/9(In9)
  In71/1 -> row_8/8(In8)
  In79/1 -> row_9/7(In7)
  In26/1 -> row_3/8(In8)
  In76/1 -> row_9/4(In4)
  In77/1 -> row_9/5(In5)
  In21/1 -> row_3/3(In3)
  In67/1 -> row_8/4(In4)
  In68/1 -> row_8/5(In5)
  In75/1 -> row_9/3(In3)
  In64/1 -> row_8/1(In1)
  In27/1 -> row_3/9(In9)
  In81/1 -> row_9/9(In9)
  In70/1 -> row_8/7(In7)
  In23/1 -> row_3/5(In5)
  In73/1 -> row_9/1(In1)
  In41/1 -> row_5/5(In5)
  In24/1 -> row_3/6(In6)
  In44/1 -> row_5/8(In8)
  In74/1 -> row_9/2(In2)
  In40/1 -> row_5/4(In4)
  In66/1 -> row_8/3(In3)
  In78/1 -> row_9/6(In6)
  In19/1 -> row_3/1(In1)
  row_1/1(Out1) -> Logical Operator/1
  row_2/1(Out1) -> Logical Operator/2
  row_3/1(Out1) -> Logical Operator/3
  row_4/1(Out1) -> Logical Operator/4
  row_5/1(Out1) -> Logical Operator/5
  row_6/1(Out1) -> Logical Operator/6
  row_7/1(Out1) -> Logical Operator/7
  row_8/1(Out1) -> Logical Operator/8
  row_9/1(Out1) -> Logical Operator/9
  Logical Operator/1 -> Out1/1

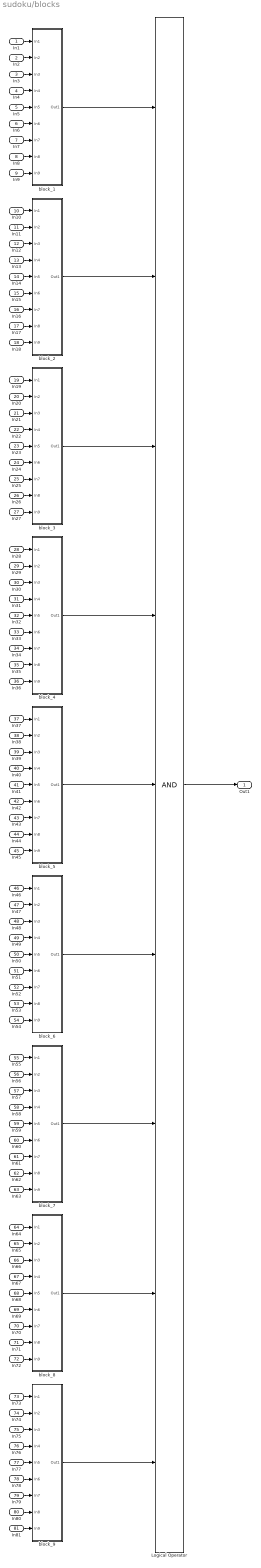
== system sudoku/blocks ==
  In1 : Inport
  In2 : Inport  Port=2
  In3 : Inport  Port=3
  In4 : Inport  Port=4
  In5 : Inport  Port=5
  In6 : Inport  Port=6
  In7 : Inport  Port=7
  In8 : Inport  Port=8
  In9 : Inport  Port=9
  In10 : Inport  Port=10
  In11 : Inport  Port=11
  In12 : Inport  Port=12
  In13 : Inport  Port=13
  In14 : Inport  Port=14
  In15 : Inport  Port=15
  In16 : Inport  Port=16
  In17 : Inport  Port=17
  In18 : Inport  Port=18
  In19 : Inport  Port=19
  In20 : Inport  Port=20
  In21 : Inport  Port=21
  In22 : Inport  Port=22
  In23 : Inport  Port=23
  In24 : Inport  Port=24
  In25 : Inport  Port=25
  In26 : Inport  Port=26
  In27 : Inport  Port=27
  In28 : Inport  Port=28
  In29 : Inport  Port=29
  In30 : Inport  Port=30
  In31 : Inport  Port=31
  In32 : Inport  Port=32
  In33 : Inport  Port=33
  In34 : Inport  Port=34
  In35 : Inport  Port=35
  In36 : Inport  Port=36
  In37 : Inport  Port=37
  In38 : Inport  Port=38
  In39 : Inport  Port=39
  In40 : Inport  Port=40
  In41 : Inport  Port=41
  In42 : Inport  Port=42
  In43 : Inport  Port=43
  In44 : Inport  Port=44
  In45 : Inport  Port=45
  In46 : Inport  Port=46
  In47 : Inport  Port=47
  In48 : Inport  Port=48
  In49 : Inport  Port=49
  In50 : Inport  Port=50
  In51 : Inport  Port=51
  In52 : Inport  Port=52
  In53 : Inport  Port=53
  In54 : Inport  Port=54
  In55 : Inport  Port=55
  In56 : Inport  Port=56
  In57 : Inport  Port=57
  In58 : Inport  Port=58
  In59 : Inport  Port=59
  In60 : Inport  Port=60
  In61 : Inport  Port=61
  In62 : Inport  Port=62
  In63 : Inport  Port=63
  In64 : Inport  Port=64
  In65 : Inport  Port=65
  In66 : Inport  Port=66
  In67 : Inport  Port=67
  In68 : Inport  Port=68
  In69 : Inport  Port=69
  In70 : Inport  Port=70
  In71 : Inport  Port=71
  In72 : Inport  Port=72
  In73 : Inport  Port=73
  In74 : Inport  Port=74
  In75 : Inport  Port=75
  In76 : Inport  Port=76
  In77 : Inport  Port=77
  In78 : Inport  Port=78
  In79 : Inport  Port=79
  In80 : Inport  Port=80
  In81 : Inport  Port=81
  Logical Operator : Logic  Inputs=9  AllPortsSameDT=off  OutDataTypeStr=boolean
  block_1 : Subsystem
  block_2 : Subsystem
  block_3 : Subsystem
  block_4 : Subsystem
  block_5 : Subsystem
  block_6 : Subsystem
  block_7 : Subsystem
  block_8 : Subsystem
  block_9 : Subsystem
  Out1 : Outport
  wires:
  In13/1 -> block_2/4(In4)
  In10/1 -> block_2/1(In1)
  In14/1 -> block_2/5(In5)
  In16/1 -> block_2/7(In7)
  In18/1 -> block_2/9(In9)
  In12/1 -> block_2/3(In3)
  In63/1 -> block_7/9(In9)
  In62/1 -> block_7/8(In8)
  In17/1 -> block_2/8(In8)
  In11/1 -> block_2/2(In2)
  In15/1 -> block_2/6(In6)
  In47/1 -> block_6/2(In2)
  In48/1 -> block_6/3(In3)
  In59/1 -> block_7/5(In5)
  In60/1 -> block_7/6(In6)
  In56/1 -> block_7/2(In2)
  In57/1 -> block_7/3(In3)
  In58/1 -> block_7/4(In4)
  In55/1 -> block_7/1(In1)
  In61/1 -> block_7/7(In7)
  In32/1 -> block_4/5(In5)
  In33/1 -> block_4/6(In6)
  In28/1 -> block_4/1(In1)
  In2/1 -> block_1/2(In2)
  In4/1 -> block_1/4(In4)
  In8/1 -> block_1/8(In8)
  In9/1 -> block_1/9(In9)
  In35/1 -> block_4/8(In8)
  In34/1 -> block_4/7(In7)
  In1/1 -> block_1/1(In1)
  In6/1 -> block_1/6(In6)
  In7/1 -> block_1/7(In7)
  In49/1 -> block_6/4(In4)
  In50/1 -> block_6/5(In5)
  In51/1 -> block_6/6(In6)
  In52/1 -> block_6/7(In7)
  In53/1 -> block_6/8(In8)
  In3/1 -> block_1/3(In3)
  In54/1 -> block_6/9(In9)
  In37/1 -> block_5/1(In1)
  In46/1 -> block_6/1(In1)
  In5/1 -> block_1/5(In5)
  In38/1 -> block_5/2(In2)
  In39/1 -> block_5/3(In3)
  In36/1 -> block_4/9(In9)
  In29/1 -> block_4/2(In2)
  In30/1 -> block_4/3(In3)
  In31/1 -> block_4/4(In4)
  In65/1 -> block_8/2(In2)
  In43/1 -> block_5/7(In7)
  In72/1 -> block_8/9(In9)
  In69/1 -> block_8/6(In6)
  In20/1 -> block_3/2(In2)
  In25/1 -> block_3/7(In7)
  In80/1 -> block_9/8(In8)
  In42/1 -> block_5/6(In6)
  In22/1 -> block_3/4(In4)
  In45/1 -> block_5/9(In9)
  In71/1 -> block_8/8(In8)
  In79/1 -> block_9/7(In7)
  In26/1 -> block_3/8(In8)
  In76/1 -> block_9/4(In4)
  In77/1 -> block_9/5(In5)
  In21/1 -> block_3/3(In3)
  In67/1 -> block_8/4(In4)
  In68/1 -> block_8/5(In5)
  In75/1 -> block_9/3(In3)
  In64/1 -> block_8/1(In1)
  In27/1 -> block_3/9(In9)
  In81/1 -> block_9/9(In9)
  In70/1 -> block_8/7(In7)
  In23/1 -> block_3/5(In5)
  In73/1 -> block_9/1(In1)
  In41/1 -> block_5/5(In5)
  In24/1 -> block_3/6(In6)
  In44/1 -> block_5/8(In8)
  In74/1 -> block_9/2(In2)
  In40/1 -> block_5/4(In4)
  In66/1 -> block_8/3(In3)
  In78/1 -> block_9/6(In6)
  In19/1 -> block_3/1(In1)
  block_1/1(Out1) -> Logical Operator/1
  block_2/1(Out1) -> Logical Operator/2
  block_3/1(Out1) -> Logical Operator/3
  block_4/1(Out1) -> Logical Operator/4
  block_5/1(Out1) -> Logical Operator/5
  block_6/1(Out1) -> Logical Operator/6
  block_7/1(Out1) -> Logical Operator/7
  block_8/1(Out1) -> Logical Operator/8
  block_9/1(Out1) -> Logical Operator/9
  Logical Operator/1 -> Out1/1

== system sudoku/bounds ==
  In1 : Inport
  Assumption : sldvlib/Objectives and Constraints/Assumption  enabled=on  customAVTBlockType=Assumption  intervals=true  initial=off  dispValues=on  outEnabled=on
      settings: AttributesFormatString=%<intervals>
  Logical Operator : Logic  AllPortsSameDT=off  OutDataTypeStr=boolean
  geq : RelationalOperator  Operator=<=  OutDataTypeStr=boolean
  lb : Constant  OutDataTypeStr=int8
  leq : RelationalOperator  Operator=<=  OutDataTypeStr=boolean
  ub : Constant  Value=9  OutDataTypeStr=int8
  wires:
  In1/1 -> geq/1, leq/2
  geq/1 -> Logical Operator/2
  ub/1 -> geq/2
  leq/1 -> Logical Operator/1
  Logical Operator/1 -> Assumption/1
  lb/1 -> leq/1

== system sudoku/bounds1 ==
  In1 : Inport
  Assumption : sldvlib/Objectives and Constraints/Assumption  enabled=on  customAVTBlockType=Assumption  intervals=true  initial=off  dispValues=on  outEnabled=on
      settings: AttributesFormatString=%<intervals>
  Logical Operator : Logic  AllPortsSameDT=off  OutDataTypeStr=boolean
  geq : RelationalOperator  Operator=<=  OutDataTypeStr=boolean
  lb : Constant  OutDataTypeStr=int8
  leq : RelationalOperator  Operator=<=  OutDataTypeStr=boolean
  ub : Constant  Value=9  OutDataTypeStr=int8
  wires:
  In1/1 -> geq/1, leq/2
  geq/1 -> Logical Operator/2
  ub/1 -> geq/2
  leq/1 -> Logical Operator/1
  Logical Operator/1 -> Assumption/1
  lb/1 -> leq/1

== system sudoku/bounds10 ==
  In1 : Inport
  Assumption : sldvlib/Objectives and Constraints/Assumption  enabled=on  customAVTBlockType=Assumption  intervals=true  initial=off  dispValues=on  outEnabled=on
      settings: AttributesFormatString=%<intervals>
  Logical Operator : Logic  AllPortsSameDT=off  OutDataTypeStr=boolean
  geq : RelationalOperator  Operator=<=  OutDataTypeStr=boolean
  lb : Constant  OutDataTypeStr=int8
  leq : RelationalOperator  Operator=<=  OutDataTypeStr=boolean
  ub : Constant  Value=9  OutDataTypeStr=int8
  wires:
  In1/1 -> geq/1, leq/2
  geq/1 -> Logical Operator/2
  ub/1 -> geq/2
  leq/1 -> Logical Operator/1
  Logical Operator/1 -> Assumption/1
  lb/1 -> leq/1

== system sudoku/bounds11 ==
  In1 : Inport
  Assumption : sldvlib/Objectives and Constraints/Assumption  enabled=on  customAVTBlockType=Assumption  intervals=true  initial=off  dispValues=on  outEnabled=on
      settings: AttributesFormatString=%<intervals>
  Logical Operator : Logic  AllPortsSameDT=off  OutDataTypeStr=boolean
  geq : RelationalOperator  Operator=<=  OutDataTypeStr=boolean
  lb : Constant  OutDataTypeStr=int8
  leq : RelationalOperator  Operator=<=  OutDataTypeStr=boolean
  ub : Constant  Value=9  OutDataTypeStr=int8
  wires:
  In1/1 -> geq/1, leq/2
  geq/1 -> Logical Operator/2
  ub/1 -> geq/2
  leq/1 -> Logical Operator/1
  Logical Operator/1 -> Assumption/1
  lb/1 -> leq/1

== system sudoku/bounds12 ==
  In1 : Inport
  Assumption : sldvlib/Objectives and Constraints/Assumption  enabled=on  customAVTBlockType=Assumption  intervals=true  initial=off  dispValues=on  outEnabled=on
      settings: AttributesFormatString=%<intervals>
  Logical Operator : Logic  AllPortsSameDT=off  OutDataTypeStr=boolean
  geq : RelationalOperator  Operator=<=  OutDataTypeStr=boolean
  lb : Constant  OutDataTypeStr=int8
  leq : RelationalOperator  Operator=<=  OutDataTypeStr=boolean
  ub : Constant  Value=9  OutDataTypeStr=int8
  wires:
  In1/1 -> geq/1, leq/2
  geq/1 -> Logical Operator/2
  ub/1 -> geq/2
  leq/1 -> Logical Operator/1
  Logical Operator/1 -> Assumption/1
  lb/1 -> leq/1

== system sudoku/bounds13 ==
  In1 : Inport
  Assumption : sldvlib/Objectives and Constraints/Assumption  enabled=on  customAVTBlockType=Assumption  intervals=true  initial=off  dispValues=on  outEnabled=on
      settings: AttributesFormatString=%<intervals>
  Logical Operator : Logic  AllPortsSameDT=off  OutDataTypeStr=boolean
  geq : RelationalOperator  Operator=<=  OutDataTypeStr=boolean
  lb : Constant  OutDataTypeStr=int8
  leq : RelationalOperator  Operator=<=  OutDataTypeStr=boolean
  ub : Constant  Value=9  OutDataTypeStr=int8
  wires:
  In1/1 -> geq/1, leq/2
  geq/1 -> Logical Operator/2
  ub/1 -> geq/2
  leq/1 -> Logical Operator/1
  Logical Operator/1 -> Assumption/1
  lb/1 -> leq/1

== system sudoku/bounds14 ==
  In1 : Inport
  Assumption : sldvlib/Objectives and Constraints/Assumption  enabled=on  customAVTBlockType=Assumption  intervals=true  initial=off  dispValues=on  outEnabled=on
      settings: AttributesFormatString=%<intervals>
  Logical Operator : Logic  AllPortsSameDT=off  OutDataTypeStr=boolean
  geq : RelationalOperator  Operator=<=  OutDataTypeStr=boolean
  lb : Constant  OutDataTypeStr=int8
  leq : RelationalOperator  Operator=<=  OutDataTypeStr=boolean
  ub : Constant  Value=9  OutDataTypeStr=int8
  wires:
  In1/1 -> geq/1, leq/2
  geq/1 -> Logical Operator/2
  ub/1 -> geq/2
  leq/1 -> Logical Operator/1
  Logical Operator/1 -> Assumption/1
  lb/1 -> leq/1

== system sudoku/bounds15 ==
  In1 : Inport
  Assumption : sldvlib/Objectives and Constraints/Assumption  enabled=on  customAVTBlockType=Assumption  intervals=true  initial=off  dispValues=on  outEnabled=on
      settings: AttributesFormatString=%<intervals>
  Logical Operator : Logic  AllPortsSameDT=off  OutDataTypeStr=boolean
  geq : RelationalOperator  Operator=<=  OutDataTypeStr=boolean
  lb : Constant  OutDataTypeStr=int8
  leq : RelationalOperator  Operator=<=  OutDataTypeStr=boolean
  ub : Constant  Value=9  OutDataTypeStr=int8
  wires:
  In1/1 -> geq/1, leq/2
  geq/1 -> Logical Operator/2
  ub/1 -> geq/2
  leq/1 -> Logical Operator/1
  Logical Operator/1 -> Assumption/1
  lb/1 -> leq/1

== system sudoku/bounds16 ==
  In1 : Inport
  Assumption : sldvlib/Objectives and Constraints/Assumption  enabled=on  customAVTBlockType=Assumption  intervals=true  initial=off  dispValues=on  outEnabled=on
      settings: AttributesFormatString=%<intervals>
  Logical Operator : Logic  AllPortsSameDT=off  OutDataTypeStr=boolean
  geq : RelationalOperator  Operator=<=  OutDataTypeStr=boolean
  lb : Constant  OutDataTypeStr=int8
  leq : RelationalOperator  Operator=<=  OutDataTypeStr=boolean
  ub : Constant  Value=9  OutDataTypeStr=int8
  wires:
  In1/1 -> geq/1, leq/2
  geq/1 -> Logical Operator/2
  ub/1 -> geq/2
  leq/1 -> Logical Operator/1
  Logical Operator/1 -> Assumption/1
  lb/1 -> leq/1

== system sudoku/bounds17 ==
  In1 : Inport
  Assumption : sldvlib/Objectives and Constraints/Assumption  enabled=on  customAVTBlockType=Assumption  intervals=true  initial=off  dispValues=on  outEnabled=on
      settings: AttributesFormatString=%<intervals>
  Logical Operator : Logic  AllPortsSameDT=off  OutDataTypeStr=boolean
  geq : RelationalOperator  Operator=<=  OutDataTypeStr=boolean
  lb : Constant  OutDataTypeStr=int8
  leq : RelationalOperator  Operator=<=  OutDataTypeStr=boolean
  ub : Constant  Value=9  OutDataTypeStr=int8
  wires:
  In1/1 -> geq/1, leq/2
  geq/1 -> Logical Operator/2
  ub/1 -> geq/2
  leq/1 -> Logical Operator/1
  Logical Operator/1 -> Assumption/1
  lb/1 -> leq/1

== system sudoku/bounds18 ==
  In1 : Inport
  Assumption : sldvlib/Objectives and Constraints/Assumption  enabled=on  customAVTBlockType=Assumption  intervals=true  initial=off  dispValues=on  outEnabled=on
      settings: AttributesFormatString=%<intervals>
  Logical Operator : Logic  AllPortsSameDT=off  OutDataTypeStr=boolean
  geq : RelationalOperator  Operator=<=  OutDataTypeStr=boolean
  lb : Constant  OutDataTypeStr=int8
  leq : RelationalOperator  Operator=<=  OutDataTypeStr=boolean
  ub : Constant  Value=9  OutDataTypeStr=int8
  wires:
  In1/1 -> geq/1, leq/2
  geq/1 -> Logical Operator/2
  ub/1 -> geq/2
  leq/1 -> Logical Operator/1
  Logical Operator/1 -> Assumption/1
  lb/1 -> leq/1

== system sudoku/bounds19 ==
  In1 : Inport
  Assumption : sldvlib/Objectives and Constraints/Assumption  enabled=on  customAVTBlockType=Assumption  intervals=true  initial=off  dispValues=on  outEnabled=on
      settings: AttributesFormatString=%<intervals>
  Logical Operator : Logic  AllPortsSameDT=off  OutDataTypeStr=boolean
  geq : RelationalOperator  Operator=<=  OutDataTypeStr=boolean
  lb : Constant  OutDataTypeStr=int8
  leq : RelationalOperator  Operator=<=  OutDataTypeStr=boolean
  ub : Constant  Value=9  OutDataTypeStr=int8
  wires:
  In1/1 -> geq/1, leq/2
  geq/1 -> Logical Operator/2
  ub/1 -> geq/2
  leq/1 -> Logical Operator/1
  Logical Operator/1 -> Assumption/1
  lb/1 -> leq/1
